simulink model "Fuzzy"  (R2023b)
settings: Solver=ode23t  StartTime=0.0  StopTime=14  FixedStep=0.0001  MaxStep=0.05  RelTol=1e-3  EnableMultiTasking=on
model workspace (MAT data in the model file):
  DCMotor_J = 0.0946866703633
  DCMotor_K = 0.477771340295
  DCMotor_Kf = 0.921434142151
  DCMotor_L = 0.000316454712175
  DCMotor_R = 4.99938152603
  Ts = 0.1
  dFilt = [1 -0.1202]
  nFilt = [0.4399 0.4399]
undefined symbols (not defined in the file): X, Y, Z
libraries: sm_lib x488, fl_lib x150, nesl_utility x56, ee_lib x42, slpidlib x12, fuzblock x6, SignalEditorBlockLib x1
(part 1 of 12)
settings Model: Creator=The MathWorks, Inc.  LastModifiedBy=d8436
settings SolverCC: AlgebraicLoopSolver=TrustRegion
settings DataIOCC: LimitDataPoints=on  SaveFormat=Array  InspectSignalLogs=on  SaveTime=off  ReturnWorkspaceOutputs=off
settings OptimizationCC: ReuseModelBlockBuffer=off  ExpressionDepthLimit=2147483647  LifeSpan=inf
settings DebuggingCC: UnderspecifiedInitializationDetection=Classic  MergeDetectMultiDrivingBlocksExec=none  FcnCallInpInsideContextMsg=warning  UnconnectedInputMsg=warning  UnconnectedOutputMsg=warning  UnconnectedLineMsg=warning  StateNameClashWarn=warning  SFUnexpectedBacktrackingDiag=warning  SFNoUnconditionalDefaultTransitionDiag=warning  SFExecutionAtInitializationDiag=none  ArithmeticOperatorsInVariantConditions=warning
settings HardwareCC: ProdBitPerPointer=32  ProdBitPerSizeT=32  ProdBitPerPtrDiffT=32  ProdLargestAtomicFloat=None  ProdIntDivRoundTo=Undefined  ProdEndianess=Unspecified  ProdWordSize=32  ProdHWDeviceType=32-bit Generic
settings ModelReferenceCC: EnableRefExpFcnMdlSchedulingChecks=on  PropagateSignalLabelsOutOfModel=off
settings SFSimCC: SimUseLocalCustomCode=off  CustomCodeUndefinedFunction=UseInterfaceOnly
settings RTWCC: RTWUseLocalCustomCode=off
settings CodeAppCC: StateflowObjectComments=on
settings GRTTargetCC: TargetLangStandard=C89/C90 (ANSI)  CombineOutputUpdateFcns=off  GRTInterface=on
settings ConfigComp: CovMetricSettings=dw  CovSaveCumulativeToWorkspaceVar=on  CovSaveSingleToWorkspaceVar=on  CovExternalEMLEnable=off  CovSFcnEnable=off
settings SimscapeCC: SimscapeNormalizeSystem=off
settings ConfigurationSet: Description=SimMechanics 2G
settings DiagnosticsConfigSet: SimMechanicsUnconnectedFramePorts=none
settings ExplorerConfigSet: InternalSimMechanicsExplorerSettings="<ExplorerConfiguration><canonicalview>planar_xy</canonicalview><AnimationSetting><BasePlaybackSpeed>1.0</BasePlaybackSpeed><PlaybackSpeedFactor>1.0</PlaybackSpeedFactor></AnimationSetting><TilePanel><TileInfo><Tiles Columns=\"1\" Count=\"1\" Rows=\"1\"><Column Weight=\"1\"/><Row Weight=\"1\"/><Tile Height=\"1\" Width=\"1\" X=\"0\" Y=\"0\"/></Tiles></TileInfo><SceneInfo><SceneViewer><BGColor><R>0.800000011920928955</R><G>0.800000011920928955</G><B>0.800000011920928955</B></BGColor><Camera><DoPerspective>off</DoPerspective><Position><X>0.307524879443026977</X><Y>0.579228365631063946</Y><Z>0.356513057442465364</Z></Position><Center><X>-0.0337723867490332744</X><Y>0.237931099438984189</Y><Z>0.0152157912503931205</Z></Center><Up><X>-0.408248290463863073</X><Y>0.816496580927726145</Y><Z>-0.408248290463863073</Z></Up><ViewLimDist>1</ViewLimDist><YLim>0.22321517040744418</YLim><XLim>0.362893073821357937</XLim></Camera></SceneViewer></SceneInfo></TilePanel><MechEditorPanel><Cameras/><GfxPanelCameraMap/><VideoCreator><PlaybackSpeedRatio>1.0</PlaybackSpeedRatio><FrameRate>30</FrameRate><VideoFormat>Motion JPEG AVI</VideoFormat><FrameSize>auto</FrameSize></VideoCreator></MechEditorPanel></ExplorerConfiguration>"

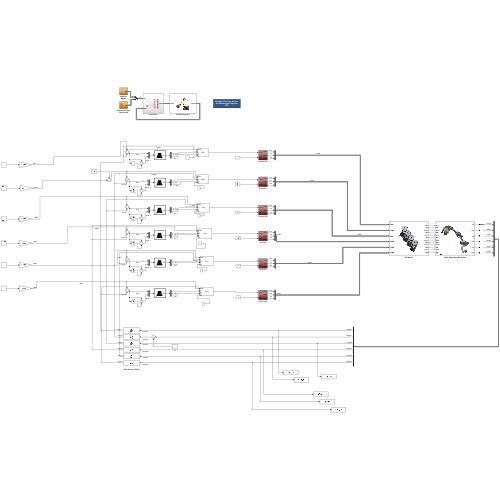
[thumbnail: Simulink's stored preview of the top-level diagram]
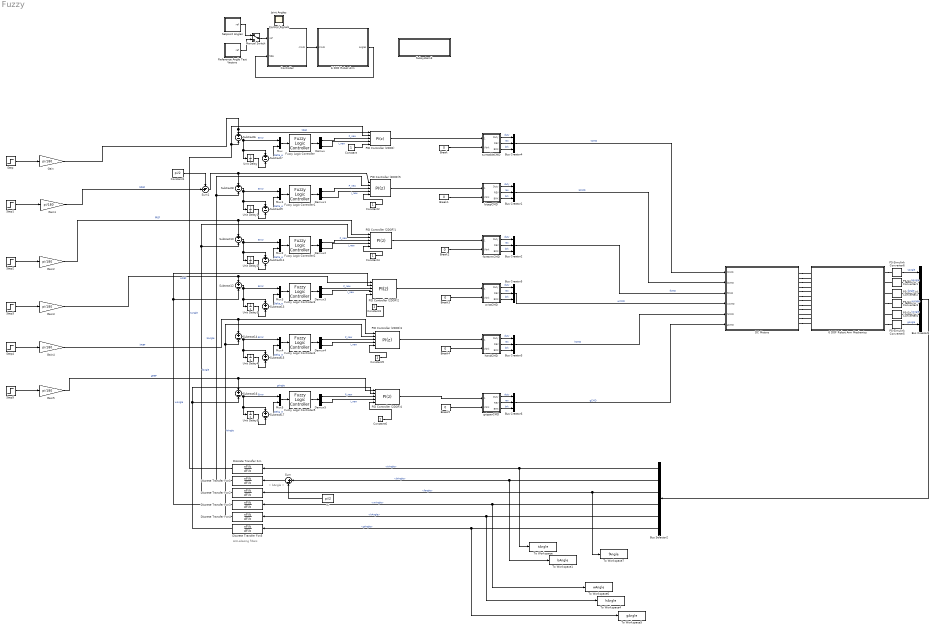
== system Fuzzy ==
  note: < bAngle >
  note: Anti-aliasing filters
  6 DOF Robot Arm : Subsystem
      mask Display: image('RobotArmSystem.jpg',[0.2 0.05 0.6 0.9])
  6 DOF Robot Arm Mechanics : Subsystem
      mask Display: image('RobotArm_Mechanics.jpg',[0.1 0 0.8 1])
  Break{,1..5} (6 alike) : Constant  Value=0
  Bus Creator{1..6} (6 alike) : BusCreator  Inputs=3
  Bus Creator8 : BusCreator  Inputs=6
  Bus Selector2 : BusSelector  OutputSignals=tAngle,bAngle,fangle,wAngle,hAngle,gAngle
  Constant{,2..6} (6 alike) : Constant
  Constant1 : Constant  Value=pi/2
  Controller : Subsystem
  DC Motors : Subsystem
      mask Display: image('MultiServos.jpg',[0.25 0.1 0.5 0.8])
  Demux{,1..5} (6 alike) : Demux  Outputs=2
  Discrete Transfer Fcn{,1..5} (6 alike) : DiscreteTransferFcn  Numerator=nFilt  Denominator=dFilt  SampleTime=Ts
  Fuzzy Logic Controller{,1..5} (6 alike) : fuzblock/Fuzzy Logic  Controller  FIS=PI_Fuzzy  OutputSampleNumber=101  DataType=double  FuzzifiedInputs=off  RuleFiringStrengths=off  RuleOutputs=off  AggregatedOutputs=off  SimulateUsing=Interpreted execution  OutOfRangeInputValueMessage=warning  NoRuleFiredMessage=warning  EmptyOutputFuzzySetMessage=warning
  Gain{,1..5} (6 alike) : Gain  Gain=pi/180
  IC : Constant  Value=pi/2
  Manual Switch : ManualSwitch
  Mux{,1..5} (6 alike) : Mux  Inputs=2
  PID Controller (2DOF){,1..5} (6 alike) : slpidlib/PID Controller (2DOF)  Controller=PI  Form=Parallel  TimeDomain=Discrete-time  UseExternalTs=off  SampleTime=Ts  IntegratorMethod=Forward Euler  FilterMethod=Forward Euler  ControllerParametersSource=external  P=1  I=1  UseKiTs=off  D=0  N=100  UseFilter=on  b=1  c=1  TunerSelectOption=Transfer Function Based (PID Tuner App)  InitialConditionSource=internal  InitialConditionForIntegrator=0  InitialConditionForFilter=0  DifferentiatorICPrevScaledInput=0  ExternalReset=none  TrackingMode=off  Kt=1  LimitOutput=off  SatLimitsSource=internal  UpperSaturationLimit=inf  LowerSaturationLimit=-inf  LinearizeAsGain=on  AntiWindupMode=none  Kb=1  LimitIntegrator=off  UpperIntegratorSaturationLimit=inf  LowerIntegratorSaturationLimit=-inf  POutMin=[]  POutMax=[]  IOutMin=[]  IOutMax=[]  DOutMin=[]  DOutMax=[]  NOutMin=[]  NOutMax=[]  bOutMin=[]  bOutMax=[]  cOutMin=[]  cOutMax=[]  SumOutMin=[]  SumOutMax=[]  SaturationOutMin=[]  SaturationOutMax=[]  PParamMin=[]  PParamMax=[]  IParamMin=[]  IParamMax=[]  DParamMin=[]  DParamMax=[]  NParamMin=[]  NParamMax=[]  bParamMin=[]  bParamMax=[]  cParamMin=[]  cParamMax=[]  KbParamMin=[]  KbParamMax=[]  KtParamMin=[]  KtParamMax=[]  KbOutMin=[]  KbOutMax=[]  KtOutMin=[]  KtOutMax=[]  IntegratorOutMin=[]  IntegratorOutMax=[]  FilterOutMin=[]  FilterOutMax=[]  SumI1OutMin=[]  SumI1OutMax=[]  SumI2OutMin=[]  SumI2OutMax=[]  SumI3OutMin=[]  SumI3OutMax=[]  SumI4OutMin=[]  SumI4OutMax=[]  SumDOutMin=[]  SumDOutMax=[]  Sum1OutMin=[]  Sum1OutMax=[]  Sum2OutMin=[]  Sum2OutMax=[]  Sum3OutMin=[]  Sum3OutMax=[]  DifferentiatorOutMin=[]  DifferentiatorOutMax=[]  FilterDiffOutCoefMin=[]  FilterDiffOutCoefMax=[]  ReciprocalOutMin=[]  ReciprocalOutMax=[]  SumDenOutMin=[]  SumDenOutMax=[]  SumNumOutMin=[]  SumNumOutMax=[]  DivideOutMin=[]  DivideOutMax=[]  UdiffTsProdOutMin=[]  UdiffTsProdOutMax=[]  NTsProdOutMin=[]  NTsProdOutMax=[]  UintegralTsProdOutMin=[]  UintegralTsProdOutMax=[]  UngainTsProdOutMin=[]  UngainTsProdOutMax=[]  ClampingZeroOutDataTypeStr=Inherit: Inherit via back propagation  ClampingZeroOutMin=[]  ClampingZeroOutMax=[]  FilterDenConstantOutDataTypeStr=Inherit: Inherit via back propagation  FilterDenConstantOutMin=[]  FilterDenConstantOutMax=[]  PCopyOutDataTypeStr=Inherit: Inherit via back propagation  PCopyOutMin=[]  PCopyOutMax=[]  NCopyOutDataTypeStr=Inherit: Inherit via back propagation  NCopyOutMin=[]  NCopyOutMax=[]  IntegratorContinuousStateAttributes=''  IntegratorStateMustResolveToSignalObject=off  IntegratorRTWStateStorageClass=Auto  FilterContinuousStateAttributes=''  FilterStateMustResolveToSignalObject=off  FilterRTWStateStorageClass=Auto  ParallelPVariant=ExternalParameters  IdealPVariant=Disabled  IVariant=ExternalParameters  DVariant=Disabled  bVariant=ExternalParameters  cVariant=Disabled  IntegratorVariant=Discrete  SatVariant=Disabled  AWVariant=Passthrough  PCopyVariant=Disabled  TRVariant=Disabled  FdbkBlocksVariant=Forward  IdealPFdbkVariant=Disabled  SatFdbkVariant=Disabled  DerivativeFilterVariant=Disabled  NVariant=Disabled  NCopyVariant=Disabled_SignalSpec  FilterICVariant=Disabled  IntegratorICVariant=InternalICs  ExternalResetVariant=Disabled  TRSumVariant=Passthrough  SumFdbkVariant=Disabled  SumVariant=Sum_PI  TsampFilterVariant=InternalTs  TsampNgainVariant=Passthrough  TsampIntegralVariant=Disabled_SignalSpec  ExternalSaturationOutDataTypeStr=Inherit: Same as second input
  PS-Simulink Converter{1..6} (6 alike) : nesl_utility/PS-Simulink Converter  PhysicalDomain=network_engine_domain  SubClassName=ps_output  LeftPortType=input  RightPortType=output  PseudoPeriodic=off  Frequencies=[]  VectorFormat=1-D array  Unit=rad  AffineConversion=off
  Reference Angle Test Vectors : Subsystem
  Setpoint Angles : Subsystem
  Step : Step  Time=0  After=60  SampleTime=Ts
  Step1 : Step  Time=0  Before=90  After=80  SampleTime=Ts
  Step2 : Step  Time=0  After=60  SampleTime=Ts
  Step3 : Step  Time=0  After=90  SampleTime=Ts
  Step4 : Step  Time=0  After=90  SampleTime=Ts
  Step5 : Step  Time=0  After=60  SampleTime=Ts
  Subsystem3 : Subsystem
      mask init:
      | % Get current simulation mode
      | vizStatus = get_param(gcs,'SimMechanicsOpenEditorOnUpdate');
      | 
      | if strcmp(vizStatus,'on')
      |     viz = 'OFF';
      | else
      |     viz = 'ON';
      | end
      settings: OpenFcn=|
      | % Get current SimMechanics Explorer status
      | vizStatus = get_param(gcs ,'SimMechanicsOpenEditorOnUpdate');
      | 
      | if strcmp(vizStatus,'on')
      | % Set SimMechanics Explorer status to OFF
      |      set_param(gcs,'SimMechanicsOpenEditorOnUpdate','off');
      |      set_param(gcb,'BackgroundColor','[0.4706, 0.4706, 0.4706]');
      |      set_param(gcs,'SimulationCommand','update');
      | else
      | % Set SimMechanics Explorer status to ON
      |      set_param(gcs,'SimMechanicsOpenEditorOnUpdate','on');
      |      set_param(gcb,'BackgroundColor','[0.1961, 0.3412, 0.5176]')
      |      set_param(gcs,'SimulationCommand','update');
      | end
      mask Display:
      | color('white')
      | text(0.5,0.65,'Double-click here to turn\nthe Mechanics Explorer',...
      |     'horizontalAlignment','center',...
      |     'verticalAlignment','middle');
      | text(0.5,0.25,viz,...
      |     'horizontalAlignment','center',...
      |     'verticalAlignment','middle')
  Subtract{6..17} (12 alike) : Sum  Inputs=+-
  Sum : Sum  Inputs=|+-
  Sum1 : Sum  Inputs=-+|
  To Workspace : ToWorkspace  VariableName=tAngle  SampleTime=Ts
      settings: Save2DSignal=2-D array (concatenate along first dimension)
  To Workspace1 : ToWorkspace  VariableName=bAngle  SampleTime=Ts
      settings: Save2DSignal=2-D array (concatenate along first dimension)
  To Workspace4 : ToWorkspace  VariableName=hAngle  SampleTime=Ts
      settings: Save2DSignal=2-D array (concatenate along first dimension)
  To Workspace5 : ToWorkspace  VariableName=gAngle  SampleTime=Ts
      settings: Save2DSignal=2-D array (concatenate along first dimension)
  To Workspace6 : ToWorkspace  VariableName=wAngle  SampleTime=Ts
      settings: Save2DSignal=2-D array (concatenate along first dimension)
  To Workspace7 : ToWorkspace  VariableName=fAngle  SampleTime=Ts
      settings: Save2DSignal=2-D array (concatenate along first dimension)
  Unit Delay{,1..5} (6 alike) : UnitDelay  SampleTime=-1  HasFrameUpgradeWarning=on
  bicepCMD : Subsystem
  forearmCMD : Subsystem
  gripperCMD : Subsystem
  handCMD : Subsystem
  turntableCMD : Subsystem
  wristCMD : Subsystem
  Control Signals : Scope
  Joint Angles : Scope
  wires:
  Controller/1(cmds) -> 6 DOF Robot Arm/1(cmds)
  6 DOF Robot Arm/1(angles) -> Controller/2(fdbk)
  Manual Switch/1 -> Controller/1(ref)
  Reference Angle Test Vectors/1(ref) -> Manual Switch/2
  Setpoint Angles/1(ref) -> Manual Switch/1
  Gain1/1 -> Sum1/2  "bREF"
  Gain2/1 -> PID Controller (2DOF)1/1, Subtract10/1  "fREF"
  Gain5/1 -> PID Controller (2DOF)4/1, Subtract16/1  "gREF"
  Gain4/1 -> PID Controller (2DOF)3/1, Subtract14/1  "hREF"
  Gain/1 -> PID Controller (2DOF)/1, Subtract6/1  "tREF"
  Gain3/1 -> PID Controller (2DOF)2/1, Subtract12/1  "wREF"
  Constant1/1 -> Sum1/1
  Bus Creator1/1 -> DC Motors/2(bCMD)  "bCMD"
  wristCMD/3(BRK) -> Bus Creator5/3  "brk"
  forearmCMD/2(REV) -> Bus Creator2/2  "rev"
  Bus Creator2/1 -> DC Motors/3(fCMD)  "fCMD"
  gripperCMD/1(Duty) -> Bus Creator6/1  "duty"
  Bus Creator6/1 -> DC Motors/6(gCMD)  "gCMD"
  Break3/1 -> wristCMD/2(Vbrk)
  forearmCMD/3(BRK) -> Bus Creator2/3  "brk"
  wristCMD/2(REV) -> Bus Creator5/2  "rev"
  turntableCMD/3(BRK) -> Bus Creator4/3  "brk"
  gripperCMD/2(REV) -> Bus Creator6/2  "rev"
  gripperCMD/3(BRK) -> Bus Creator6/3  "brk"
  Break5/1 -> gripperCMD/2(Vbrk)
  Bus Creator4/1 -> DC Motors/1(tCMD)  "tCMD"
  bicepCMD/2(REV) -> Bus Creator1/2  "rev"
  Bus Creator3/1 -> DC Motors/5(hCMD)  "hCMD"
  Bus Creator5/1 -> DC Motors/4(wCMD)  "wCMD"
  Break/1 -> turntableCMD/2(Vbrk)
  handCMD/1(Duty) -> Bus Creator3/1  "duty"
  forearmCMD/1(Duty) -> Bus Creator2/1  "duty"
  handCMD/2(REV) -> Bus Creator3/2  "rev"
  turntableCMD/1(Duty) -> Bus Creator4/1  "duty"
  handCMD/3(BRK) -> Bus Creator3/3  "brk"
  bicepCMD/3(BRK) -> Bus Creator1/3  "brk"
  Break1/1 -> bicepCMD/2(Vbrk)
  Break2/1 -> forearmCMD/2(Vbrk)
  turntableCMD/2(REV) -> Bus Creator4/2  "rev"
  Break4/1 -> handCMD/2(Vbrk)
  wristCMD/1(Duty) -> Bus Creator5/1  "duty"
  PS-Simulink Converter5/1 -> Bus Creator8/6  "gAngle"
  PS-Simulink Converter3/1 -> Bus Creator8/4  "wAngle"
  PS-Simulink Converter2/1 -> Bus Creator8/3  "fangle"
  PS-Simulink Converter4/1 -> Bus Creator8/5  "hAngle"
  Sum/1 -> Discrete Transfer Fcn1/1
  Bus Selector2/2 -> To Workspace1/1, Sum/1  "<bAngle>"
  Bus Selector2/6 -> To Workspace5/1, Discrete Transfer Fcn5/1  "<gAngle>"
  Bus Selector2/1 -> To Workspace/1, Discrete Transfer Fcn/1  "<tAngle>"
  Bus Selector2/5 -> To Workspace4/1, Discrete Transfer Fcn4/1  "<hAngle>"
  IC/1 -> Sum/2
  Bus Selector2/4 -> To Workspace6/1, Discrete Transfer Fcn3/1  "<wAngle>"
  Bus Creator8/1 -> Bus Selector2/1
  Bus Selector2/3 -> To Workspace7/1, Discrete Transfer Fcn2/1  "<fangle>"
  PID Controller (2DOF)/1 -> turntableCMD/1(Vcmd)
  Discrete Transfer Fcn/1 -> Subtract6/2, PID Controller (2DOF)/2  "tAngle"
  Constant/1 -> PID Controller (2DOF)/5
  Constant2/1 -> PID Controller (2DOF)5/5
  PID Controller (2DOF)5/1 -> bicepCMD/1(Vcmd)
  Sum1/1 -> PID Controller (2DOF)5/1, Subtract8/1
  Constant4/1 -> PID Controller (2DOF)1/5
  PID Controller (2DOF)1/1 -> forearmCMD/1(Vcmd)
  Constant3/1 -> PID Controller (2DOF)2/5
  PID Controller (2DOF)2/1 -> wristCMD/1(Vcmd)
  PID Controller (2DOF)3/1 -> handCMD/1(Vcmd)
  Constant5/1 -> PID Controller (2DOF)3/5
  PID Controller (2DOF)4/1 -> gripperCMD/1(Vcmd)
  Constant6/1 -> PID Controller (2DOF)4/5
  PS-Simulink Converter1/1 -> Bus Creator8/2  "bAngle"
  PS-Simulink Converter6/1 -> Bus Creator8/1  "tAngle"
  bicepCMD/1(Duty) -> Bus Creator1/1  "duty"
  Step/1 -> Gain/1
  Step1/1 -> Gain1/1
  Step2/1 -> Gain2/1
  Step3/1 -> Gain3/1
  Step4/1 -> Gain4/1
  Step5/1 -> Gain5/1
  Subtract6/1 -> Mux/1, Subtract7/1, Unit Delay/1  "Error"
  Unit Delay/1 -> Subtract7/2
  Subtract7/1 -> Mux/2  "Delta_e"
  Mux/1 -> Fuzzy Logic Controller/1
  Fuzzy Logic Controller/1 -> Demux/1
  Demux/1 -> PID Controller (2DOF)/3  "P_new"
  Demux/2 -> PID Controller (2DOF)/4  "I_new"
  Discrete Transfer Fcn1/1 -> Subtract8/2, PID Controller (2DOF)5/2  "bAngle"
  Demux1/2 -> PID Controller (2DOF)5/4  "I_new"
  Subtract8/1 -> Mux1/1, Subtract9/1, Unit Delay1/1  "Error"
  Mux1/1 -> Fuzzy Logic Controller1/1
  Unit Delay1/1 -> Subtract9/2
  Demux1/1 -> PID Controller (2DOF)5/3  "P_new"
  Fuzzy Logic Controller1/1 -> Demux1/1
  Subtract9/1 -> Mux1/2  "Delta_e"
  Discrete Transfer Fcn2/1 -> Subtract10/2, PID Controller (2DOF)1/2  "fAngle"
  Demux2/2 -> PID Controller (2DOF)1/4  "I_new"
  Subtract10/1 -> Mux2/1, Subtract11/1, Unit Delay2/1  "Error"
  Mux2/1 -> Fuzzy Logic Controller2/1
  Unit Delay2/1 -> Subtract11/2
  Demux2/1 -> PID Controller (2DOF)1/3  "P_new"
  Fuzzy Logic Controller2/1 -> Demux2/1
  Subtract11/1 -> Mux2/2  "Delta_e"
  Discrete Transfer Fcn3/1 -> PID Controller (2DOF)2/2, Subtract12/2  "wAngle"
  Demux3/2 -> PID Controller (2DOF)2/4  "I_new"
  Subtract12/1 -> Mux3/1, Subtract13/1, Unit Delay3/1  "Error"
  Mux3/1 -> Fuzzy Logic Controller3/1
  Unit Delay3/1 -> Subtract13/2
  Demux3/1 -> PID Controller (2DOF)2/3  "P_new"
  Fuzzy Logic Controller3/1 -> Demux3/1
  Subtract13/1 -> Mux3/2  "Delta_e"
  Discrete Transfer Fcn4/1 -> Subtract14/2, PID Controller (2DOF)3/2  "hAngle"
  Demux4/2 -> PID Controller (2DOF)3/4  "I_new"
  Subtract14/1 -> Mux4/1, Subtract15/1, Unit Delay4/1  "Error"
  Mux4/1 -> Fuzzy Logic Controller4/1
  Unit Delay4/1 -> Subtract15/2
  Demux4/1 -> PID Controller (2DOF)3/3  "P_new"
  Fuzzy Logic Controller4/1 -> Demux4/1
  Subtract15/1 -> Mux4/2  "Delta_e"
  Discrete Transfer Fcn5/1 -> PID Controller (2DOF)4/2, Subtract16/2  "gAngle"
  Demux5/2 -> PID Controller (2DOF)4/4  "I_new"
  Subtract16/1 -> Mux5/1, Subtract17/1, Unit Delay5/1  "Error"
  Mux5/1 -> Fuzzy Logic Controller5/1
  Unit Delay5/1 -> Subtract17/2
  Demux5/1 -> PID Controller (2DOF)4/3  "P_new"
  Fuzzy Logic Controller5/1 -> Demux5/1
  Subtract17/1 -> Mux5/2  "Delta_e"
  connections:
  6 DOF Robot Arm Mechanics/RConn4 -- PS-Simulink Converter3/LConn1
  DC Motors/RConn1 -- 6 DOF Robot Arm Mechanics/LConn1
  PS-Simulink Converter2/LConn1 -- 6 DOF Robot Arm Mechanics/RConn3
  PS-Simulink Converter4/LConn1 -- 6 DOF Robot Arm Mechanics/RConn5
  DC Motors/RConn5 -- 6 DOF Robot Arm Mechanics/LConn5
  DC Motors/RConn2 -- 6 DOF Robot Arm Mechanics/LConn2
  DC Motors/RConn12 -- 6 DOF Robot Arm Mechanics/LConn12
  DC Motors/RConn11 -- 6 DOF Robot Arm Mechanics/LConn11
  DC Motors/RConn8 -- 6 DOF Robot Arm Mechanics/LConn8
  DC Motors/RConn7 -- 6 DOF Robot Arm Mechanics/LConn7
  DC Motors/RConn9 -- 6 DOF Robot Arm Mechanics/LConn9
  DC Motors/RConn6 -- 6 DOF Robot Arm Mechanics/LConn6
  DC Motors/RConn3 -- 6 DOF Robot Arm Mechanics/LConn3
  6 DOF Robot Arm Mechanics/RConn6 -- PS-Simulink Converter5/LConn1
  DC Motors/RConn4 -- 6 DOF Robot Arm Mechanics/LConn4
  6 DOF Robot Arm Mechanics/LConn10 -- DC Motors/RConn10
  PS-Simulink Converter1/LConn1 -- 6 DOF Robot Arm Mechanics/RConn2
  6 DOF Robot Arm Mechanics/RConn1 -- PS-Simulink Converter6/LConn1

== system Fuzzy/6 DOF Robot Arm ==
  note: 6 DOF Robot Arm Manipulator - Electrical + Mechanical Plant Model
  cmds : Inport
  6 DOF Robot Arm Mechanics : Subsystem
      mask Display: image('RobotArm_Mechanics.jpg',[0.1 0 0.8 1])
  Bus Creator : BusCreator  Inputs=6
  Bus Selector : BusSelector  OutputSignals=tCMD,bCMD,fCMD,wCMD,hCMD,gCMD
  DC Motors : Subsystem
      mask Display: image('MultiServos.jpg',[0.25 0.1 0.5 0.8])
  PS-Simulink Converter{,1..5} (6 alike) : nesl_utility/PS-Simulink Converter  PhysicalDomain=network_engine_domain  SubClassName=ps_output  LeftPortType=input  RightPortType=output  PseudoPeriodic=off  Frequencies=[]  VectorFormat=1-D array  Unit=rad  AffineConversion=off
  angles : Outport  VectorParamsAs1DForOutWhenUnconnected=off
  wires:
  Bus Creator/1 -> angles/1
  PS-Simulink Converter2/1 -> Bus Creator/3  "fAngle"
  PS-Simulink Converter5/1 -> Bus Creator/6  "gAngle"
  PS-Simulink Converter/1 -> Bus Creator/1  "tAngle"
  PS-Simulink Converter1/1 -> Bus Creator/2  "bAngle"
  PS-Simulink Converter3/1 -> Bus Creator/4  "wAngle"
  PS-Simulink Converter4/1 -> Bus Creator/5  "hAngle"
  Bus Selector/6 -> DC Motors/6(gCMD)  "<gCMD>"
  Bus Selector/3 -> DC Motors/3(fCMD)  "<fCMD>"
  Bus Selector/4 -> DC Motors/4(wCMD)  "<wCMD>"
  Bus Selector/2 -> DC Motors/2(bCMD)  "<bCMD>"
  Bus Selector/5 -> DC Motors/5(hCMD)  "<hCMD>"
  Bus Selector/1 -> DC Motors/1(tCMD)  "<tCMD>"
  cmds/1 -> Bus Selector/1
  connections:
  PS-Simulink Converter2/LConn1 -- 6 DOF Robot Arm Mechanics/RConn3
  DC Motors/RConn7 -- 6 DOF Robot Arm Mechanics/LConn7
  DC Motors/RConn8 -- 6 DOF Robot Arm Mechanics/LConn8
  DC Motors/RConn6 -- 6 DOF Robot Arm Mechanics/LConn6
  PS-Simulink Converter/LConn1 -- 6 DOF Robot Arm Mechanics/RConn1
  DC Motors/RConn2 -- 6 DOF Robot Arm Mechanics/LConn2
  DC Motors/RConn5 -- 6 DOF Robot Arm Mechanics/LConn5
  DC Motors/RConn11 -- 6 DOF Robot Arm Mechanics/LConn11
  DC Motors/RConn12 -- 6 DOF Robot Arm Mechanics/LConn12
  DC Motors/RConn9 -- 6 DOF Robot Arm Mechanics/LConn9
  DC Motors/RConn3 -- 6 DOF Robot Arm Mechanics/LConn3
  DC Motors/RConn4 -- 6 DOF Robot Arm Mechanics/LConn4
  PS-Simulink Converter1/LConn1 -- 6 DOF Robot Arm Mechanics/RConn2
  PS-Simulink Converter4/LConn1 -- 6 DOF Robot Arm Mechanics/RConn5
  6 DOF Robot Arm Mechanics/RConn6 -- PS-Simulink Converter5/LConn1
  6 DOF Robot Arm Mechanics/RConn4 -- PS-Simulink Converter3/LConn1
  DC Motors/RConn10 -- 6 DOF Robot Arm Mechanics/LConn10
  DC Motors/RConn1 -- 6 DOF Robot Arm Mechanics/LConn1

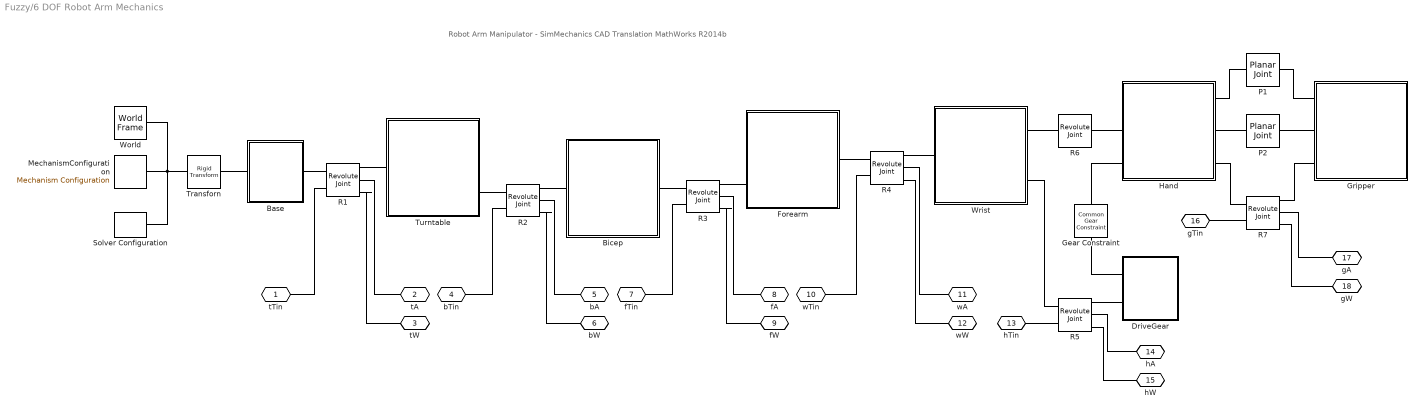
== system Fuzzy/6 DOF Robot Arm Mechanics ==
  note: Robot Arm Manipulator - SimMechanics CAD Translation
      | MathWorks R2014b
  Base : Subsystem
      mask Display: image('Base.jpg',[0.25,0.25,0.5,0.5])
  Bicep : Subsystem
      mask Display: image('Bicep.jpg')
  DriveGear : Subsystem
      mask Display: image('DriveGear.jpg',[0.2,0.2,0.6,0.6])
  Forearm : Subsystem
      mask Display: image('Forearm.jpg')
  Gear Constraint : sm_lib/Gears and Couplings/Gears/Common Gear Constraint  GearType=External  SpecificationType=CenterDistanceRatio  CenterDistance=39.8888296  CenterDistanceUnits=mm  GearRatio=1.0  BaseGearRadius=10.0  BaseGearRadiusUnits=cm  FollGearRadius=10.0  FollGearRadiusUnits=cm  AssemblyGearRotation=Free
  Gripper : Subsystem
      mask Display: image('Gripper.jpg',[0.1,0.1,0.8,0.8])
  Hand : Subsystem
      mask Display: image('Hand.jpg',[0.1,0.1,0.8,0.8])
  MechanismConfiguration : sm_lib/Utilities/Mechanism Configuration  UniformGravity=Constant  GravityVector=[0 -9.81 0]  GravityVectorUnits=m/s^2  LinearizationDelta=0.001  JointModeTransitionNonlinearIterations=2
  P1 : sm_lib/Joints/Planar Joint  JointMode=Normal  SenseConstraintForce=off  SenseConstraintForceX=off  SenseConstraintForceY=off  SenseConstraintForceZ=off  SenseConstraintTorque=off  SenseConstraintTorqueX=off  SenseConstraintTorqueY=off  SenseConstraintTorqueZ=off  SenseTotalForce=off  SenseTotalForceX=off  SenseTotalForceY=off  SenseTotalForceZ=off  SenseTotalTorque=off  SenseTotalTorqueX=off  SenseTotalTorqueY=off  SenseTotalTorqueZ=off  CompositeWrenchDir=FollowerOnBase  CompositeWrenchFrame=BaseFrame  PxEquilibriumPosition=0  PxEquilibriumPositionUnits=m  PxSpringStiffness=0  PxSpringStiffnessUnits=N/m  PxDampingCoefficient=0  PxDampingCoefficientUnits=s*N/m  PxTorqueActuationMode=NoTorque  PxMotionActuationMode=ComputedMotion  PxSensePosition=off  PxSenseVelocity=off  PxSenseAcceleration=off  PxSenseTorqueForce=off  PxSenseLowerLimitTorqueForce=off  PxSenseUpperLimitTorqueForce=off  PxLowerLimitSpecify=off  PxLowerLimitBound=-1  PxLowerLimitBoundUnits=m  PxLowerLimitStiffness=1e6  PxLowerLimitStiffnessUnits=N/m  PxLowerLimitDamping=1e3  PxLowerLimitDampingUnits=N/(m/s)  PxLowerLimitTransitionRegionWidth=1e-4  PxLowerLimitTransitionRegionWidthUnits=m  PxUpperLimitSpecify=off  PxUpperLimitBound=1  PxUpperLimitBoundUnits=m  PxUpperLimitStiffness=1e6  PxUpperLimitStiffnessUnits=N/m  PxUpperLimitDamping=1e3  PxUpperLimitDampingUnits=N/(m/s)  PxUpperLimitTransitionRegionWidth=1e-4  PxUpperLimitTransitionRegionWidthUnits=m  PxPositionTargetSpecify=off  PxPositionTargetPriority=High  PxPositionTargetValue=0  PxPositionTargetValueUnits=m  PxVelocityTargetSpecify=off  PxVelocityTargetPriority=High  PxVelocityTargetValue=0  PxVelocityTargetValueUnits=m/s  PyEquilibriumPosition=0  PyEquilibriumPositionUnits=m  PySpringStiffness=0  PySpringStiffnessUnits=N/m  PyDampingCoefficient=0  PyDampingCoefficientUnits=s*N/m  PyTorqueActuationMode=NoTorque  PyMotionActuationMode=ComputedMotion  PySensePosition=off  PySenseVelocity=off  PySenseAcceleration=off  PySenseTorqueForce=off  PySenseLowerLimitTorqueForce=off  PySenseUpperLimitTorqueForce=off  PyLowerLimitSpecify=off  PyLowerLimitBound=-1  PyLowerLimitBoundUnits=m  PyLowerLimitStiffness=1e6  PyLowerLimitStiffnessUnits=N/m  PyLowerLimitDamping=1e3  PyLowerLimitDampingUnits=N/(m/s)  PyLowerLimitTransitionRegionWidth=1e-4  PyLowerLimitTransitionRegionWidthUnits=m  PyUpperLimitSpecify=off  PyUpperLimitBound=1  PyUpperLimitBoundUnits=m  PyUpperLimitStiffness=1e6  PyUpperLimitStiffnessUnits=N/m  PyUpperLimitDamping=1e3  PyUpperLimitDampingUnits=N/(m/s)  PyUpperLimitTransitionRegionWidth=1e-4  PyUpperLimitTransitionRegionWidthUnits=m  PyPositionTargetSpecify=off  PyPositionTargetPriority=High  PyPositionTargetValue=0  PyPositionTargetValueUnits=m  PyVelocityTargetSpecify=off  PyVelocityTargetPriority=High  PyVelocityTargetValue=0  PyVelocityTargetValueUnits=m/s  RzEquilibriumPosition=0  RzEquilibriumPositionUnits=rad  RzSpringStiffness=0  RzSpringStiffnessUnits=m*N/rad  RzDampingCoefficient=0  RzDampingCoefficientUnits=m*s*N/rad  RzTorqueActuationMode=NoTorque  RzMotionActuationMode=ComputedMotion  RzSensePosition=off  RzSenseVelocity=off  RzSenseAcceleration=off  RzSenseTorqueForce=off  RzSenseLowerLimitTorqueForce=off  RzSenseUpperLimitTorqueForce=off  RzLowerLimitSpecify=off  RzLowerLimitBound=-90  RzLowerLimitBoundUnits=deg  RzLowerLimitStiffness=1e4  RzLowerLimitStiffnessUnits=N*m/deg  RzLowerLimitDamping=10  RzLowerLimitDampingUnits=N*m/(deg/s)  RzLowerLimitTransitionRegionWidth=0.1  RzLowerLimitTransitionRegionWidthUnits=deg  RzUpperLimitSpecify=off  RzUpperLimitBound=90  RzUpperLimitBoundUnits=deg  RzUpperLimitStiffness=1e4  RzUpperLimitStiffnessUnits=N*m/deg  RzUpperLimitDamping=10  RzUpperLimitDampingUnits=N*m/(deg/s)  RzUpperLimitTransitionRegionWidth=0.1  RzUpperLimitTransitionRegionWidthUnits=deg  RzPositionTargetSpecify=off  RzPositionTargetPriority=High  RzPositionTargetValue=0  RzPositionTargetValueUnits=deg  RzVelocityTargetSpecify=off  RzVelocityTargetPriority=High  RzVelocityTargetValue=0  RzVelocityTargetValueUnits=deg/s
  P2 : sm_lib/Joints/Planar Joint  JointMode=Normal  SenseConstraintForce=off  SenseConstraintForceX=off  SenseConstraintForceY=off  SenseConstraintForceZ=off  SenseConstraintTorque=off  SenseConstraintTorqueX=off  SenseConstraintTorqueY=off  SenseConstraintTorqueZ=off  SenseTotalForce=off  SenseTotalForceX=off  SenseTotalForceY=off  SenseTotalForceZ=off  SenseTotalTorque=off  SenseTotalTorqueX=off  SenseTotalTorqueY=off  SenseTotalTorqueZ=off  CompositeWrenchDir=FollowerOnBase  CompositeWrenchFrame=BaseFrame  PxEquilibriumPosition=0  PxEquilibriumPositionUnits=m  PxSpringStiffness=0  PxSpringStiffnessUnits=N/m  PxDampingCoefficient=0  PxDampingCoefficientUnits=s*N/m  PxTorqueActuationMode=NoTorque  PxMotionActuationMode=ComputedMotion  PxSensePosition=off  PxSenseVelocity=off  PxSenseAcceleration=off  PxSenseTorqueForce=off  PxSenseLowerLimitTorqueForce=off  PxSenseUpperLimitTorqueForce=off  PxLowerLimitSpecify=off  PxLowerLimitBound=-1  PxLowerLimitBoundUnits=m  PxLowerLimitStiffness=1e6  PxLowerLimitStiffnessUnits=N/m  PxLowerLimitDamping=1e3  PxLowerLimitDampingUnits=N/(m/s)  PxLowerLimitTransitionRegionWidth=1e-4  PxLowerLimitTransitionRegionWidthUnits=m  PxUpperLimitSpecify=off  PxUpperLimitBound=1  PxUpperLimitBoundUnits=m  PxUpperLimitStiffness=1e6  PxUpperLimitStiffnessUnits=N/m  PxUpperLimitDamping=1e3  PxUpperLimitDampingUnits=N/(m/s)  PxUpperLimitTransitionRegionWidth=1e-4  PxUpperLimitTransitionRegionWidthUnits=m  PxPositionTargetSpecify=off  PxPositionTargetPriority=High  PxPositionTargetValue=0  PxPositionTargetValueUnits=m  PxVelocityTargetSpecify=off  PxVelocityTargetPriority=High  PxVelocityTargetValue=0  PxVelocityTargetValueUnits=m/s  PyEquilibriumPosition=0  PyEquilibriumPositionUnits=m  PySpringStiffness=0  PySpringStiffnessUnits=N/m  PyDampingCoefficient=0  PyDampingCoefficientUnits=s*N/m  PyTorqueActuationMode=NoTorque  PyMotionActuationMode=ComputedMotion  PySensePosition=off  PySenseVelocity=off  PySenseAcceleration=off  PySenseTorqueForce=off  PySenseLowerLimitTorqueForce=off  PySenseUpperLimitTorqueForce=off  PyLowerLimitSpecify=off  PyLowerLimitBound=-1  PyLowerLimitBoundUnits=m  PyLowerLimitStiffness=1e6  PyLowerLimitStiffnessUnits=N/m  PyLowerLimitDamping=1e3  PyLowerLimitDampingUnits=N/(m/s)  PyLowerLimitTransitionRegionWidth=1e-4  PyLowerLimitTransitionRegionWidthUnits=m  PyUpperLimitSpecify=off  PyUpperLimitBound=1  PyUpperLimitBoundUnits=m  PyUpperLimitStiffness=1e6  PyUpperLimitStiffnessUnits=N/m  PyUpperLimitDamping=1e3  PyUpperLimitDampingUnits=N/(m/s)  PyUpperLimitTransitionRegionWidth=1e-4  PyUpperLimitTransitionRegionWidthUnits=m  PyPositionTargetSpecify=off  PyPositionTargetPriority=High  PyPositionTargetValue=0  PyPositionTargetValueUnits=m  PyVelocityTargetSpecify=off  PyVelocityTargetPriority=High  PyVelocityTargetValue=0  PyVelocityTargetValueUnits=m/s  RzEquilibriumPosition=0  RzEquilibriumPositionUnits=rad  RzSpringStiffness=0  RzSpringStiffnessUnits=m*N/rad  RzDampingCoefficient=0  RzDampingCoefficientUnits=m*s*N/rad  RzTorqueActuationMode=NoTorque  RzMotionActuationMode=ComputedMotion  RzSensePosition=off  RzSenseVelocity=off  RzSenseAcceleration=off  RzSenseTorqueForce=off  RzSenseLowerLimitTorqueForce=off  RzSenseUpperLimitTorqueForce=off  RzLowerLimitSpecify=off  RzLowerLimitBound=-90  RzLowerLimitBoundUnits=deg  RzLowerLimitStiffness=1e4  RzLowerLimitStiffnessUnits=N*m/deg  RzLowerLimitDamping=10  RzLowerLimitDampingUnits=N*m/(deg/s)  RzLowerLimitTransitionRegionWidth=0.1  RzLowerLimitTransitionRegionWidthUnits=deg  RzUpperLimitSpecify=off  RzUpperLimitBound=90  RzUpperLimitBoundUnits=deg  RzUpperLimitStiffness=1e4  RzUpperLimitStiffnessUnits=N*m/deg  RzUpperLimitDamping=10  RzUpperLimitDampingUnits=N*m/(deg/s)  RzUpperLimitTransitionRegionWidth=0.1  RzUpperLimitTransitionRegionWidthUnits=deg  RzPositionTargetSpecify=off  RzPositionTargetPriority=High  RzPositionTargetValue=0  RzPositionTargetValueUnits=deg  RzVelocityTargetSpecify=off  RzVelocityTargetPriority=High  RzVelocityTargetValue=0  RzVelocityTargetValueUnits=deg/s
  R{1,3..5,7} (5 alike) : sm_lib/Joints/Revolute Joint  JointMode=Normal  SenseConstraintForce=off  SenseConstraintForceX=off  SenseConstraintForceY=off  SenseConstraintForceZ=off  SenseConstraintTorque=off  SenseConstraintTorqueX=off  SenseConstraintTorqueY=off  SenseConstraintTorqueZ=off  SenseTotalForce=off  SenseTotalForceX=off  SenseTotalForceY=off  SenseTotalForceZ=off  SenseTotalTorque=off  SenseTotalTorqueX=off  SenseTotalTorqueY=off  SenseTotalTorqueZ=off  CompositeWrenchDir=FollowerOnBase  CompositeWrenchFrame=BaseFrame  EquilibriumPosition=0  EquilibriumPositionUnits=rad  SpringStiffness=0  SpringStiffnessUnits=m*N/rad  DampingCoefficient=0  DampingCoefficientUnits=m*s*N/rad  TorqueActuationMode=InputTorque  MotionActuationMode=ComputedMotion  SensePosition=on  SenseVelocity=on  SenseAcceleration=off  SenseTorqueForce=off  SenseLowerLimitTorqueForce=off  SenseUpperLimitTorqueForce=off  LowerLimitSpecify=off  LowerLimitBound=-90  LowerLimitBoundUnits=deg  LowerLimitStiffness=1e4  LowerLimitStiffnessUnits=N*m/deg  LowerLimitDamping=10  LowerLimitDampingUnits=N*m/(deg/s)  LowerLimitTransitionRegionWidth=0.1  LowerLimitTransitionRegionWidthUnits=deg  UpperLimitSpecify=off  UpperLimitBound=90  UpperLimitBoundUnits=deg  UpperLimitStiffness=1e4  UpperLimitStiffnessUnits=N*m/deg  UpperLimitDamping=10  UpperLimitDampingUnits=N*m/(deg/s)  UpperLimitTransitionRegionWidth=0.1  UpperLimitTransitionRegionWidthUnits=deg  PositionTargetSpecify=on  PositionTargetPriority=High  PositionTargetValue=0  PositionTargetValueUnits=deg  VelocityTargetSpecify=on  VelocityTargetPriority=High  VelocityTargetValue=0  VelocityTargetValueUnits=deg/s
  R2 : sm_lib/Joints/Revolute Joint  JointMode=Normal  SenseConstraintForce=off  SenseConstraintForceX=off  SenseConstraintForceY=off  SenseConstraintForceZ=off  SenseConstraintTorque=off  SenseConstraintTorqueX=off  SenseConstraintTorqueY=off  SenseConstraintTorqueZ=off  SenseTotalForce=off  SenseTotalForceX=off  SenseTotalForceY=off  SenseTotalForceZ=off  SenseTotalTorque=off  SenseTotalTorqueX=off  SenseTotalTorqueY=off  SenseTotalTorqueZ=off  CompositeWrenchDir=FollowerOnBase  CompositeWrenchFrame=BaseFrame  EquilibriumPosition=0  EquilibriumPositionUnits=rad  SpringStiffness=0  SpringStiffnessUnits=m*N/rad  DampingCoefficient=0  DampingCoefficientUnits=m*s*N/rad  TorqueActuationMode=InputTorque  MotionActuationMode=ComputedMotion  SensePosition=on  SenseVelocity=on  SenseAcceleration=off  SenseTorqueForce=off  SenseLowerLimitTorqueForce=off  SenseUpperLimitTorqueForce=off  LowerLimitSpecify=off  LowerLimitBound=-90  LowerLimitBoundUnits=deg  LowerLimitStiffness=1e4  LowerLimitStiffnessUnits=N*m/deg  LowerLimitDamping=10  LowerLimitDampingUnits=N*m/(deg/s)  LowerLimitTransitionRegionWidth=0.1  LowerLimitTransitionRegionWidthUnits=deg  UpperLimitSpecify=off  UpperLimitBound=90  UpperLimitBoundUnits=deg  UpperLimitStiffness=1e4  UpperLimitStiffnessUnits=N*m/deg  UpperLimitDamping=10  UpperLimitDampingUnits=N*m/(deg/s)  UpperLimitTransitionRegionWidth=0.1  UpperLimitTransitionRegionWidthUnits=deg  PositionTargetSpecify=on  PositionTargetPriority=High  PositionTargetValue=90  PositionTargetValueUnits=deg  VelocityTargetSpecify=on  VelocityTargetPriority=High  VelocityTargetValue=0  VelocityTargetValueUnits=deg/s
  R6 : sm_lib/Joints/Revolute Joint  JointMode=Normal  SenseConstraintForce=off  SenseConstraintForceX=off  SenseConstraintForceY=off  SenseConstraintForceZ=off  SenseConstraintTorque=off  SenseConstraintTorqueX=off  SenseConstraintTorqueY=off  SenseConstraintTorqueZ=off  SenseTotalForce=off  SenseTotalForceX=off  SenseTotalForceY=off  SenseTotalForceZ=off  SenseTotalTorque=off  SenseTotalTorqueX=off  SenseTotalTorqueY=off  SenseTotalTorqueZ=off  CompositeWrenchDir=FollowerOnBase  CompositeWrenchFrame=BaseFrame  EquilibriumPosition=0  EquilibriumPositionUnits=rad  SpringStiffness=0  SpringStiffnessUnits=m*N/rad  DampingCoefficient=0  DampingCoefficientUnits=m*s*N/rad  TorqueActuationMode=NoTorque  MotionActuationMode=ComputedMotion  SensePosition=off  SenseVelocity=off  SenseAcceleration=off  SenseTorqueForce=off  SenseLowerLimitTorqueForce=off  SenseUpperLimitTorqueForce=off  LowerLimitSpecify=off  LowerLimitBound=-90  LowerLimitBoundUnits=deg  LowerLimitStiffness=1e4  LowerLimitStiffnessUnits=N*m/deg  LowerLimitDamping=10  LowerLimitDampingUnits=N*m/(deg/s)  LowerLimitTransitionRegionWidth=0.1  LowerLimitTransitionRegionWidthUnits=deg  UpperLimitSpecify=off  UpperLimitBound=90  UpperLimitBoundUnits=deg  UpperLimitStiffness=1e4  UpperLimitStiffnessUnits=N*m/deg  UpperLimitDamping=10  UpperLimitDampingUnits=N*m/(deg/s)  UpperLimitTransitionRegionWidth=0.1  UpperLimitTransitionRegionWidthUnits=deg  PositionTargetSpecify=on  PositionTargetPriority=High  PositionTargetValue=-90  PositionTargetValueUnits=deg  VelocityTargetSpecify=on  VelocityTargetPriority=High  VelocityTargetValue=0  VelocityTargetValueUnits=deg/s
  Solver Configuration : nesl_utility/Solver Configuration  PhysicalDomain=network_engine_domain  SubClassName=solver  LeftPortType=input  RightPortType=generic  Tones=[]  Harmonics=[]  SimulateNoise=off  Profile=off  UseLocalSampling=off  EnableSwitchedLinearOptims=on  FrequencyDomain=off  UseCCode=off  RelTol=0.001  AbsTol=1e-06  MinStep=1e-09  ToWorkspace=off  RevertToSquareIcSolve=off  NumHomotopyIterations=100  PhasorMode=off  PhasorModeNumHarmonics=1  ConsistencySolver=NEWTON_FTOL  IndexReductionMethod=DerivativeReplacement  DoDC=off  ResidualTolerance=1e-09  ConsistencyTolSource=GLOBAL  ConsistencyAbsTol=0.001  ConsistencyRelTol=0.001  ConsistencyTolFactor=0.001  UseLocalSolver=off  LocalSolverChoice=NE_BACKWARD_EULER_ADVANCER  ResolveIndetEquations=on  FunctionEvalNumThread=1  LocalSolverSampleTime=0.001  DoFixedCost=off  MaxNonlinIter=3  MaxModeIter=2  ComputeImpulses=off  ImpulseIterations=2  LinearAlgebra=Sparse  LinearAlgebraNumThread=0  EquationFormulation=NE_TIME_EF  DelaysMemoryBudget=1024  AutomaticFiltering=on  FilteringTimeConstant=0.001  PartitionStorageMethod=AS_NEEDED  PartitionMemoryBudget=1024  PartitionMethod=FAST  MultibodyUseLocalSolver=off  MultibodyLocalSolverChoice=ODE1  MultibodyLocalSolverSampleTime=0.001
  Transforn : sm_lib/Frames and Transforms/Rigid Transform  TranslationMethod=None  TranslationStandardOffset=0  TranslationStandardOffsetUnits=m  TranslationStandardAxis=+Z  TranslationCartesianOffset=[0 0 0]  TranslationCartesianOffsetUnits=m  TranslationROffset=0  TranslationROffsetUnits=m  TranslationZOffset=0  TranslationZOffsetUnits=m  TranslationThetaOffset=0  TranslationThetaOffsetUnits=deg  RotationMethod=None  RotationAngleUnits=deg  RotationStandardAxis=+Z  RotationAngle=0.0  RotationArbitraryAxis=[0 0 1]  FollAlignAxisA=+X  BaseAlignAxisA=+Y  FollAlignAxisB=+Y  BaseAlignAxisB=+Z  RotationSequenceAxes=FollowerAxes  RotationSequence=XYX  RotationSequenceAngles=[0 0 0]  RotationSequenceAnglesUnits=deg  RotationMatrix=[1 0 0; 0 1 0; 0 0 1]  Quaternion=[1 0 0 0]
  Turntable : Subsystem
      mask Display: image('Turntable.jpg')
  World : sm_lib/Frames and Transforms/World Frame
  Wrist : Subsystem
      mask Display: image('Wrist.jpg')
  tTin : PMIOPort  Side=Left
  tA : PMIOPort  Port=2  Side=Right
  tW : PMIOPort  Port=3  Side=Left
  bTin : PMIOPort  Port=4  Side=Left
  bA : PMIOPort  Port=5  Side=Right
  bW : PMIOPort  Port=6  Side=Left
  fTin : PMIOPort  Port=7  Side=Left
  fA : PMIOPort  Port=8  Side=Right
  fW : PMIOPort  Port=9  Side=Left
  wTin : PMIOPort  Port=10  Side=Left
  wA : PMIOPort  Port=11  Side=Right
  wW : PMIOPort  Port=12  Side=Left
  hTin : PMIOPort  Port=13  Side=Left
  hA : PMIOPort  Port=14  Side=Right
  hW : PMIOPort  Port=15  Side=Left
  gTin : PMIOPort  Port=16  Side=Left
  gA : PMIOPort  Port=17  Side=Right
  gW : PMIOPort  Port=18  Side=Left
  connections:
  World/RConn1 -- Transforn/LConn1 -- MechanismConfiguration/RConn1 -- Solver Configuration/RConn1
  R2/LConn1 -- Turntable/RConn2
  Gripper/LConn3 -- R7/RConn1
  Hand/RConn2 -- P2/LConn1
  Gripper/LConn2 -- P2/RConn1
  R6/LConn1 -- Wrist/RConn1
  Hand/LConn2 -- R6/RConn1
  Hand/RConn1 -- P1/LConn1
  Gripper/LConn1 -- P1/RConn1
  Forearm/RConn1 -- R4/LConn1
  R4/RConn1 -- Wrist/LConn1
  Base/LConn1 -- Transforn/RConn1
  Bicep/LConn1 -- R2/RConn1
  Bicep/RConn1 -- R3/LConn1
  Forearm/LConn2 -- R3/RConn1
  R5/LConn1 -- Wrist/RConn2
  DriveGear/LConn2 -- R5/RConn1
  Base/RConn1 -- R1/LConn1
  R1/RConn1 -- Turntable/LConn1
  Hand/RConn3 -- R7/LConn1
  tTin/RConn1 -- R1/LConn2
  bTin/RConn1 -- R2/LConn2
  fTin/RConn1 -- R3/LConn2
  wTin/RConn1 -- R4/LConn2
  hTin/RConn1 -- R5/LConn2
  gTin/RConn1 -- R7/LConn2
  Gear Constraint/LConn1 -- DriveGear/LConn1
  Gear Constraint/RConn1 -- Hand/LConn3
  R1/RConn2 -- tA/RConn1
  R1/RConn3 -- tW/RConn1
  R2/RConn2 -- bA/RConn1
  R2/RConn3 -- bW/RConn1
  R3/RConn2 -- fA/RConn1
  R3/RConn3 -- fW/RConn1
  R4/RConn2 -- wA/RConn1
  R4/RConn3 -- wW/RConn1
  R5/RConn2 -- hA/RConn1
  R5/RConn3 -- hW/RConn1
  R7/RConn2 -- gA/RConn1
  R7/RConn3 -- gW/RConn1
